simulink model "model"  (R2014b)
settings: Solver=ode45  StartTime=0.0  StopTime=10.0  RelTol=1e-3
values from neighbouring files (symbols this model uses):
  alfa = 12    [fzad2.m]    (also in zad1.m; zad2.m)
  B = 2    [fzad2.m]    (also in zad1.m; zad2.m)
  beta = 3    [fzad2.m]    (also in zad1.m; zad2.m)
  d = 3    [fzad2.m]    (also in zad1.m; zad2.m)
  K = wektor(1)    [fzad2.m]    (also in zad1.m = 1.8; zad2.m = optymalne(1))
  Ki = 1    [fzad2.m]    (also in zad1.m = 0; zad2.m)
  Td = wektor(3)    [fzad2.m]    (also in zad1.m = 0; zad2.m = optymalne(3))
  Ti = wektor(2)    [fzad2.m]    (also in zad1.m = 3.3; zad2.m = optymalne(2))
  zadana = 5    [fzad2.m]    (also in zad1.m; zad2.m)
settings Model: Creator=Dyzio  LastModifiedBy=Dyzio

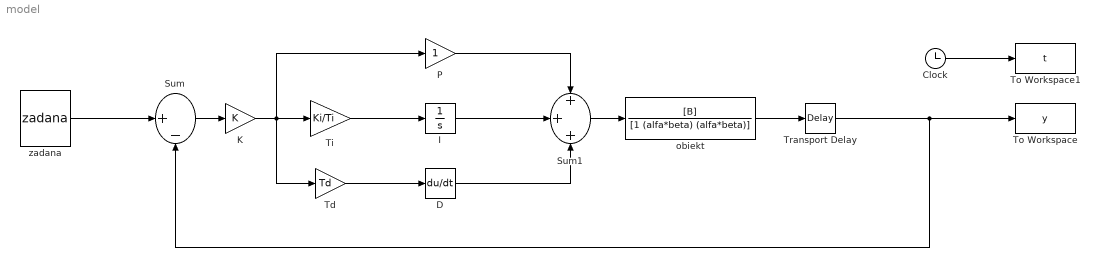
== system model ==
  Clock : Clock
  D : Derivative
  I : Integrator
  K : Gain  Gain=K
  P : Gain
  Sum : Sum  Inputs=|+-
  Sum1 : Sum  Inputs=+++
  Td : Gain  Gain=Td
  Ti : Gain  Gain=Ki/Ti
  To Workspace : ToWorkspace  VariableName=y  SampleTime=-1
  To Workspace1 : ToWorkspace  VariableName=t  SampleTime=-1
  Transport Delay : TransportDelay  DelayTime=d
  obiekt : TransferFcn  Numerator=[B]  Denominator=[1 (alfa*beta) (alfa*beta)]
  zadana : Constant  Value=zadana
  wires:
  zadana/1 -> Sum/1
  Sum/1 -> K/1
  P/1 -> Sum1/1
  K/1 -> Td/1, Ti/1, P/1
  Ti/1 -> I/1
  I/1 -> Sum1/2
  Sum1/1 -> obiekt/1
  Td/1 -> D/1
  D/1 -> Sum1/3
  obiekt/1 -> Transport Delay/1
  Clock/1 -> To Workspace1/1
  Transport Delay/1 -> Sum/2, To Workspace/1
